simulink model "sampleModel653"  (R2023a)
settings: Solver=VariableStepAuto  StartTime=0.0  StopTime=10.0  RelTol=1e-3
undefined symbols (not defined in the file): DiscIntNeverNeededParam, magnitude, Newton, Raphson
libraries: simulink x238, slpidlib x68
(part 11 of 11)

== system sampleModel653/cfblk198/cfblk15 ==
  cfblk1 : Inport
  cfblk11 : Delay
  cfblk3 : DiscreteTransferFcn
  cfblk4 : slpidlib/PID Controller (2DOF)  Controller=PID  Form=Parallel  TimeDomain=Discrete-time  UseExternalTs=off  SampleTime=-1  IntegratorMethod=Forward Euler  FilterMethod=Forward Euler  ControllerParametersSource=internal  P=1  I=1  UseKiTs=off  D=0  N=100  UseFilter=on  b=1  c=1  TunerSelectOption=Transfer Function Based (PID Tuner App)  InitialConditionSource=internal  InitialConditionForIntegrator=0  InitialConditionForFilter=0  DifferentiatorICPrevScaledInput=0  ExternalReset=none  TrackingMode=off  Kt=1  LimitOutput=off  SatLimitsSource=internal  UpperSaturationLimit=inf  LowerSaturationLimit=-inf  LinearizeAsGain=off  AntiWindupMode=none  Kb=1  LimitIntegrator=off  UpperIntegratorSaturationLimit=inf  LowerIntegratorSaturationLimit=-inf  POutMin=[]  POutMax=[]  IOutMin=[]  IOutMax=[]  DOutMin=[]  DOutMax=[]  NOutMin=[]  NOutMax=[]  bOutMin=[]  bOutMax=[]  cOutMin=[]  cOutMax=[]  SumOutMin=[]  SumOutMax=[]  SaturationOutMin=[]  SaturationOutMax=[]  PParamMin=[]  PParamMax=[]  IParamMin=[]  IParamMax=[]  DParamMin=[]  DParamMax=[]  NParamMin=[]  NParamMax=[]  bParamMin=[]  bParamMax=[]  cParamMin=[]  cParamMax=[]  KbParamMin=[]  KbParamMax=[]  KtParamMin=[]  KtParamMax=[]  KbOutMin=[]  KbOutMax=[]  KtOutMin=[]  KtOutMax=[]  IntegratorOutMin=[]  IntegratorOutMax=[]  FilterOutMin=[]  FilterOutMax=[]  SumI1OutMin=[]  SumI1OutMax=[]  SumI2OutMin=[]  SumI2OutMax=[]  SumI3OutMin=[]  SumI3OutMax=[]  SumI4OutMin=[]  SumI4OutMax=[]  SumDOutMin=[]  SumDOutMax=[]  Sum1OutMin=[]  Sum1OutMax=[]  Sum2OutMin=[]  Sum2OutMax=[]  Sum3OutMin=[]  Sum3OutMax=[]  DifferentiatorOutMin=[]  DifferentiatorOutMax=[]  FilterDiffOutCoefMin=[]  FilterDiffOutCoefMax=[]  ReciprocalOutMin=[]  ReciprocalOutMax=[]  SumDenOutMin=[]  SumDenOutMax=[]  SumNumOutMin=[]  SumNumOutMax=[]  DivideOutMin=[]  DivideOutMax=[]  UdiffTsProdOutMin=[]  UdiffTsProdOutMax=[]  NTsProdOutMin=[]  NTsProdOutMax=[]  UintegralTsProdOutMin=[]  UintegralTsProdOutMax=[]  UngainTsProdOutMin=[]  UngainTsProdOutMax=[]  ClampingZeroOutDataTypeStr=Inherit: Inherit via back propagation  ClampingZeroOutMin=[]  ClampingZeroOutMax=[]  FilterDenConstantOutDataTypeStr=Inherit: Inherit via back propagation  FilterDenConstantOutMin=[]  FilterDenConstantOutMax=[]  PCopyOutDataTypeStr=Inherit: Inherit via back propagation  PCopyOutMin=[]  PCopyOutMax=[]  NCopyOutDataTypeStr=Inherit: Inherit via back propagation  NCopyOutMin=[]  NCopyOutMax=[]  IntegratorContinuousStateAttributes=''  IntegratorStateMustResolveToSignalObject=off  IntegratorRTWStateStorageClass=Auto  FilterContinuousStateAttributes=''  FilterStateMustResolveToSignalObject=off  FilterRTWStateStorageClass=Auto  ParallelPVariant=InternalParameters  IdealPVariant=Disabled  IVariant=InternalParameters  DVariant=InternalParameters  bVariant=InternalParameters  cVariant=InternalParameters  IntegratorVariant=Discrete  SatVariant=Disabled  AWVariant=Passthrough  PCopyVariant=Disabled  TRVariant=Disabled  FdbkBlocksVariant=Forward  IdealPFdbkVariant=Disabled  SatFdbkVariant=Disabled  DerivativeFilterVariant=ForwardEulerFilter  NVariant=InternalParameters  NCopyVariant=Disabled  FilterICVariant=InternalICsFilter  IntegratorICVariant=InternalICs  ExternalResetVariant=Disabled  TRSumVariant=Passthrough  SumFdbkVariant=Disabled  SumVariant=Sum_PID  TsampFilterVariant=InternalTs  TsampNgainVariant=Passthrough  TsampIntegralVariant=Disabled_SignalSpec  ExternalSaturationOutDataTypeStr=Inherit: Same as second input
      settings: LibrarySourceBlock=simulink/Discrete/Discrete PID Controller (2DOF)
  cfblk5 : Delay
  cfblk6 : Signum
  cfblk7 : ComplexToMagnitudeAngle
  cfblk8 : Constant  Value=[-257911264.294214]  SampleTime=1
  cfblk9 : Constant  Value=[687711862.595586]  SampleTime=1
  cfblk2 : Outport
  cfblk10 : Outport  Port=2
  wires:
  cfblk1/1 -> cfblk7/1
  cfblk8/1 -> cfblk2/1
  cfblk9/1 -> cfblk10/1
  cfblk5/1 -> cfblk3/1
  cfblk6/1 -> cfblk4/2
  cfblk4/1 -> cfblk5/1
  cfblk7/1 -> cfblk6/1
  cfblk3/1 -> cfblk11/1
  cfblk11/1 -> cfblk4/1

== system sampleModel653/cfblk199/cfblk10 ==
  cfblk1 : Inport
  cfblk10 : Delay
  cfblk3 : simulink/Discrete/Transfer Fcn Real Zero  ZeroZ=0.75  ICPrevInput=0.0  DoSatur=off
  cfblk4 : DiscreteFilter
  cfblk5 : simulink/Discrete/Transfer Fcn Real Zero  ZeroZ=0.75  ICPrevInput=0.0  DoSatur=off
  cfblk6 : DiscreteStateSpace  SampleTime=-1
  cfblk7 : Sum  Inputs=+
  cfblk8 : Sum  Inputs=+-
  cfblk2 : Outport
  cfblk9 : Outport  Port=2
  wires:
  cfblk3/1 -> cfblk4/1, cfblk5/1
  cfblk1/1 -> cfblk7/1
  cfblk4/1 -> cfblk6/1, cfblk8/2
  cfblk7/1 -> cfblk9/1
  cfblk6/1 -> cfblk2/1
  cfblk5/1 -> cfblk8/1
  cfblk8/1 -> cfblk10/1
  cfblk10/1 -> cfblk3/1

== system sampleModel653/cfblk199/cfblk11 ==
  cfblk1 : Inport
  cfblk12 : Inport  Port=2
  cfblk13 : Inport  Port=3
  cfblk10 : Sum  Inputs=+
  cfblk11 : Constant  Value=[-236691372.964366]  SampleTime=1
  cfblk14 : Delay
  cfblk3 : simulink/Discrete/Transfer Fcn Real Zero  ZeroZ=0.75  ICPrevInput=0.0  DoSatur=off
  cfblk4 : Delay
  cfblk5 : Product  Inputs=*
  cfblk6 : Sqrt
  cfblk7 : MinMax  Function=max  Inputs=3
  cfblk8 : Signum
  cfblk9 : ComplexToMagnitudeAngle
  cfblk2 : Outport
  wires:
  cfblk8/1 -> cfblk2/1
  cfblk1/1 -> cfblk8/1
  cfblk10/1 -> cfblk4/1
  cfblk12/1 -> cfblk3/1
  cfblk11/1 -> cfblk7/1
  cfblk9/1 -> cfblk10/1
  cfblk3/1 -> cfblk9/1
  cfblk7/1 -> cfblk5/1
  cfblk5/1 -> cfblk6/1
  cfblk4/1 -> cfblk7/3
  cfblk6/1 -> cfblk14/1
  cfblk14/1 -> cfblk7/2

== system sampleModel653/cfblk199/cfblk12 ==
  cfblk1 : Inport
  cfblk9 : Inport  Port=2
  cfblk10 : Inport  Port=3
  cfblk3 : DiscreteTransferFcn
  cfblk4 : DiscreteStateSpace  SampleTime=-1
  cfblk5 : Bias  Bias=[-118358180.221752]  SaturateOnIntegerOverflow=off
  cfblk6 : Gain  Gain=[-289446182.790784]
  cfblk7 : PermuteDimensions
  cfblk8 : Constant  Value=[-870690986.431393]  SampleTime=1
  cfblk2 : Outport
  cfblk11 : Outport  Port=2
  wires:
  cfblk7/1 -> cfblk6/1
  cfblk4/1 -> cfblk11/1
  cfblk8/1 -> cfblk7/1
  cfblk5/1 -> cfblk3/1
  cfblk3/1 -> cfblk4/1
  cfblk1/1 -> cfblk5/1
  cfblk10/1 -> cfblk2/1

== system sampleModel653/cfblk199/cfblk9 ==
  cfblk1 : Inport
  cfblk10 : Inport  Port=2
  cfblk11 : Inport  Port=3
  cfblk13 : Delay
  cfblk14 : Delay
  cfblk3 : Delay  DelayLengthSource=Input port
      settings: InputPortMap=u0,p1
  cfblk4 : simulink/Discrete/Transfer Fcn Real Zero  ZeroZ=0.75  ICPrevInput=0.0  DoSatur=off
  cfblk5 : slpidlib/PID Controller (2DOF)  Controller=PID  Form=Parallel  TimeDomain=Discrete-time  UseExternalTs=off  SampleTime=-1  IntegratorMethod=Forward Euler  FilterMethod=Forward Euler  ControllerParametersSource=internal  P=1  I=1  UseKiTs=off  D=0  N=100  UseFilter=on  b=1  c=1  TunerSelectOption=Transfer Function Based (PID Tuner App)  InitialConditionSource=internal  InitialConditionForIntegrator=0  InitialConditionForFilter=0  DifferentiatorICPrevScaledInput=0  ExternalReset=none  TrackingMode=off  Kt=1  LimitOutput=off  SatLimitsSource=internal  UpperSaturationLimit=inf  LowerSaturationLimit=-inf  LinearizeAsGain=off  AntiWindupMode=none  Kb=1  LimitIntegrator=off  UpperIntegratorSaturationLimit=inf  LowerIntegratorSaturationLimit=-inf  POutMin=[]  POutMax=[]  IOutMin=[]  IOutMax=[]  DOutMin=[]  DOutMax=[]  NOutMin=[]  NOutMax=[]  bOutMin=[]  bOutMax=[]  cOutMin=[]  cOutMax=[]  SumOutMin=[]  SumOutMax=[]  SaturationOutMin=[]  SaturationOutMax=[]  PParamMin=[]  PParamMax=[]  IParamMin=[]  IParamMax=[]  DParamMin=[]  DParamMax=[]  NParamMin=[]  NParamMax=[]  bParamMin=[]  bParamMax=[]  cParamMin=[]  cParamMax=[]  KbParamMin=[]  KbParamMax=[]  KtParamMin=[]  KtParamMax=[]  KbOutMin=[]  KbOutMax=[]  KtOutMin=[]  KtOutMax=[]  IntegratorOutMin=[]  IntegratorOutMax=[]  FilterOutMin=[]  FilterOutMax=[]  SumI1OutMin=[]  SumI1OutMax=[]  SumI2OutMin=[]  SumI2OutMax=[]  SumI3OutMin=[]  SumI3OutMax=[]  SumI4OutMin=[]  SumI4OutMax=[]  SumDOutMin=[]  SumDOutMax=[]  Sum1OutMin=[]  Sum1OutMax=[]  Sum2OutMin=[]  Sum2OutMax=[]  Sum3OutMin=[]  Sum3OutMax=[]  DifferentiatorOutMin=[]  DifferentiatorOutMax=[]  FilterDiffOutCoefMin=[]  FilterDiffOutCoefMax=[]  ReciprocalOutMin=[]  ReciprocalOutMax=[]  SumDenOutMin=[]  SumDenOutMax=[]  SumNumOutMin=[]  SumNumOutMax=[]  DivideOutMin=[]  DivideOutMax=[]  UdiffTsProdOutMin=[]  UdiffTsProdOutMax=[]  NTsProdOutMin=[]  NTsProdOutMax=[]  UintegralTsProdOutMin=[]  UintegralTsProdOutMax=[]  UngainTsProdOutMin=[]  UngainTsProdOutMax=[]  ClampingZeroOutDataTypeStr=Inherit: Inherit via back propagation  ClampingZeroOutMin=[]  ClampingZeroOutMax=[]  FilterDenConstantOutDataTypeStr=Inherit: Inherit via back propagation  FilterDenConstantOutMin=[]  FilterDenConstantOutMax=[]  PCopyOutDataTypeStr=Inherit: Inherit via back propagation  PCopyOutMin=[]  PCopyOutMax=[]  NCopyOutDataTypeStr=Inherit: Inherit via back propagation  NCopyOutMin=[]  NCopyOutMax=[]  IntegratorContinuousStateAttributes=''  IntegratorStateMustResolveToSignalObject=off  IntegratorRTWStateStorageClass=Auto  FilterContinuousStateAttributes=''  FilterStateMustResolveToSignalObject=off  FilterRTWStateStorageClass=Auto  ParallelPVariant=InternalParameters  IdealPVariant=Disabled  IVariant=InternalParameters  DVariant=InternalParameters  bVariant=InternalParameters  cVariant=InternalParameters  IntegratorVariant=Discrete  SatVariant=Disabled  AWVariant=Passthrough  PCopyVariant=Disabled  TRVariant=Disabled  FdbkBlocksVariant=Forward  IdealPFdbkVariant=Disabled  SatFdbkVariant=Disabled  DerivativeFilterVariant=ForwardEulerFilter  NVariant=InternalParameters  NCopyVariant=Disabled  FilterICVariant=InternalICsFilter  IntegratorICVariant=InternalICs  ExternalResetVariant=Disabled  TRSumVariant=Passthrough  SumFdbkVariant=Disabled  SumVariant=Sum_PID  TsampFilterVariant=InternalTs  TsampNgainVariant=Passthrough  TsampIntegralVariant=Disabled_SignalSpec  ExternalSaturationOutDataTypeStr=Inherit: Same as second input
      settings: LibrarySourceBlock=simulink/Discrete/Discrete PID Controller (2DOF)
  cfblk6 : MinMax  Function=max  Inputs=3
  cfblk7 : Trigonometry
  cfblk8 : Sum  Inputs=+-
  cfblk9 : Constant  Value=[771825502.302683]  SampleTime=1
  cfblk2 : Outport
  cfblk12 : Outport  Port=2
  wires:
  cfblk5/1 -> cfblk4/1
  cfblk11/1 -> cfblk12/1
  cfblk10/1 -> cfblk2/1, cfblk7/1
  cfblk3/1 -> cfblk5/1
  cfblk9/1 -> cfblk8/1
  cfblk7/1 -> cfblk6/1
  cfblk1/1 -> cfblk6/2, cfblk8/2
  cfblk6/1 -> cfblk3/1
  cfblk4/1 -> cfblk13/1, cfblk14/1
  cfblk8/1 -> cfblk6/3
  cfblk13/1 -> cfblk3/2
  cfblk14/1 -> cfblk5/2

== system sampleModel653/cfblk200/cfblk6 ==
  cfblk1 : Inport
  cfblk6 : Inport  Port=2
  cfblk7 : Inport  Port=3
  cfblk3 : Gain  Gain=[-230593283.222991]
  cfblk4 : Rounding
  cfblk5 : Constant  Value=[-991824947.211989]  SampleTime=1
  cfblk2 : Outport
  wires:
  cfblk5/1 -> cfblk4/1
  cfblk7/1 -> cfblk2/1
  cfblk1/1 -> cfblk3/1

== system sampleModel653/cfblk200/cfblk8 ==
  cfblk1 : Inport
  Action Port : ActionPort  ActionPortLabel=if(u1 >= 0)
  cfblk10 : Bias  Bias=[-466356618.825275]  SaturateOnIntegerOverflow=off
  cfblk11 : Constant  Value=[-605340582.280123]  SampleTime=1
  cfblk12 : Constant  Value=[-748558413.772464]  SampleTime=1
  cfblk13 : Delay
  cfblk14 : Delay
  cfblk3 : DiscreteFir
  cfblk4 : Trigonometry
  cfblk5 : Product  Inputs=**
  cfblk6 : Product
  cfblk7 : DotProduct  OutDataTypeStr=Inherit: Inherit via internal rule
  cfblk8 : Math  Operator=transpose
  cfblk9 : Rounding
  cfblk2 : Outport
  wires:
  cfblk8/1 -> cfblk9/1
  cfblk10/1 -> cfblk3/1
  cfblk11/1 -> cfblk10/1
  cfblk1/1 -> cfblk2/1
  cfblk12/1 -> cfblk7/1
  cfblk4/1 -> cfblk7/2
  cfblk6/1 -> cfblk8/1
  cfblk9/1 -> cfblk5/2
  cfblk3/1 -> cfblk6/1
  cfblk5/1 -> cfblk4/1, cfblk14/1
  cfblk7/1 -> cfblk13/1
  cfblk13/1 -> cfblk5/1
  cfblk14/1 -> cfblk6/2

== system sampleModel653/cfblk200/cfblk9 ==
  cfblk1 : Inport
  cfblk8 : Inport  Port=2
  cfblk9 : Inport  Port=3
  Action Port : ActionPort  ActionPortLabel=else
  cfblk11 : Delay
  cfblk3 : Trigonometry
  cfblk4 : simulink/Math Operations/MinMax Running Resettable  Function=min  vinit=0.0
  cfblk5 : Product  Inputs=*
  cfblk6 : Product  Inputs=**
  cfblk7 : Constant  Value=[805638867.100519]  SampleTime=1
  cfblk2 : Outport
  cfblk10 : Outport  Port=2
  wires:
  cfblk1/1 -> cfblk2/1
  cfblk5/1 -> cfblk10/1
  cfblk8/1 -> cfblk5/1
  cfblk3/1 -> cfblk6/1
  cfblk9/1 -> cfblk6/2
  cfblk7/1 -> cfblk4/1
  cfblk6/1 -> cfblk4/2
  cfblk4/1 -> cfblk11/1
  cfblk11/1 -> cfblk3/1
